simulink model "LKAS_AutoSave_DF_20220421_1805_SW62"  (R2018b)
settings: Solver=FixedStepDiscrete  StartTime=0.0  StopTime=10.0  FixedStep=0.01  RelTol=1e-3
model workspace (MAT data in the model file):
  MCOS : class17 (value not decoded)
  MCOS : class17 (value not decoded)
  MCOS : class17 (value not decoded)
  MCOS : class17 (value not decoded)
  MCOS : class17 (value not decoded)
  MCOS : class17 (value not decoded)
  MCOS : class17 (value not decoded)
  MCOS : class17 (value not decoded)
  MCOS : class17 (value not decoded)
  MCOS : class17 (value not decoded)
  MCOS : class17 (value not decoded)
  MCOS : class17 (value not decoded)
  MCOS : class17 (value not decoded)
  MCOS : class17 (value not decoded)
  MCOS : class17 (value not decoded)
  MCOS : class17 (value not decoded)
  MCOS : class17 (value not decoded)
  MCOS : class17 (value not decoded)
  MCOS : class17 (value not decoded)
  MCOS : class17 (value not decoded)
  MCOS : class17 (value not decoded)
  MCOS : class17 (value not decoded)
  MCOS : class17 (value not decoded)
  MCOS : class17 (value not decoded)
  MCOS : class17 (value not decoded)
  MCOS : class17 (value not decoded)
  MCOS : class17 (value not decoded)
  MCOS : class17 (value not decoded)
  MCOS : class17 (value not decoded)
  MCOS : class17 (value not decoded)
  MCOS : class17 (value not decoded)
  MCOS : class17 (value not decoded)
  MCOS : class17 (value not decoded)
  MCOS : class17 (value not decoded)
  MCOS : class17 (value not decoded)
  MCOS : class17 (value not decoded)
  MCOS : class17 (value not decoded)
  MCOS : class17 (value not decoded)
  MCOS : class17 (value not decoded)
  MCOS : class17 (value not decoded)
  MCOS : class17 (value not decoded)
  MCOS : class17 (value not decoded)
  MCOS : class17 (value not decoded)
  MCOS : class17 (value not decoded)
  MCOS : class17 (value not decoded)
  MCOS : class17 (value not decoded)
  MCOS : class17 (value not decoded)
  MCOS : class17 (value not decoded)
  MCOS : class17 (value not decoded)
  MCOS : class17 (value not decoded)
  MCOS : class17 (value not decoded)
  MCOS : class17 (value not decoded)
  MCOS : class17 (value not decoded)
  MCOS : class17 (value not decoded)
  MCOS : class17 (value not decoded)
  MCOS : class17 (value not decoded)
  MCOS : class17 (value not decoded)
  MCOS : class17 (value not decoded)
  MCOS : class17 (value not decoded)
  MCOS : class17 (value not decoded)
  MCOS : class17 (value not decoded)
  MCOS : class17 (value not decoded)
  MCOS : class17 (value not decoded)
  MCOS : class17 (value not decoded)
  MCOS : class17 (value not decoded)
  MCOS : class17 (value not decoded)
  MCOS : class17 (value not decoded)
  MCOS : class17 (value not decoded)
  MCOS : class17 (value not decoded)
  MCOS : class17 (value not decoded)
  MCOS : class17 (value not decoded)
  MCOS : class17 (value not decoded)
  MCOS : class17 (value not decoded)
  MCOS : class17 (value not decoded)
  MCOS : class17 (value not decoded)
  MCOS : class17 (value not decoded)
  MCOS : class17 (value not decoded)
  MCOS : class17 (value not decoded)
  MCOS : class17 (value not decoded)
  MCOS : class17 (value not decoded)
  MCOS : class17 (value not decoded)
  MCOS : class17 (value not decoded)
  MCOS : class17 (value not decoded)
  MCOS : class17 (value not decoded)
  MCOS : class17 (value not decoded)
  MCOS : class17 (value not decoded)
  MCOS : class17 (value not decoded)
  MCOS : class17 (value not decoded)
  MCOS : class17 (value not decoded)
  MCOS : class17 (value not decoded)
  MCOS : class17 (value not decoded)
  MCOS : class17 (value not decoded)
  MCOS : class17 (value not decoded)
  MCOS : class17 (value not decoded)
  MCOS : class17 (value not decoded)
  MCOS : class17 (value not decoded)
  MCOS : class17 (value not decoded)
  MCOS : class17 (value not decoded)
  MCOS : class17 (value not decoded)
  MCOS : class17 (value not decoded)
  MCOS : class17 (value not decoded)
  MCOS : class17 (value not decoded)
  MCOS : class17 (value not decoded)
  MCOS : class17 (value not decoded)
  MCOS : class17 (value not decoded)
  MCOS : class17 (value not decoded)
  MCOS : class17 (value not decoded)
  MCOS : class17 (value not decoded)
  MCOS : class17 (value not decoded)
  MCOS : class17 (value not decoded)
undefined symbols (not defined in the file): LKA_CarWidth, LKA_SampleTime, LKA_StrRatio_C, LKA_Veh2CamL_C, LKA_Veh2CamW_C, LKA_WhlBaseL_C, LL_CompHdAg_C, LL_CompSWA_C, LL_CrvtPrvwT_C, LL_DesDvt_C, LL_DvtComp_C, LL_DvtPrvwT_C, LL_DvtSpdDet_vDvtSpdMin_C, LL_HandsOff_ExitTime, LL_HandsOff_TextTime, LL_HandsOff_WarnTime, LL_HdAgExT_C, LL_HdAgPrvwT_C, LL_LAccMax_C, LL_LAccRMax_C, LL_LDW_EarliestWarnLine_C, LL_LDW_LatestWarnLine_C, LL_LDWS_SUPPRESS_HEADING, LL_LFClb_TFC_FfCtlRatio_C, LL_LFClb_TFC_KdBalance_C, LL_LFClb_TFC_KdMaxSWA_C, LL_LFClb_TFC_KdV1_C, LL_LFClb_TFC_KdV2_C, LL_LFClb_TFC_KdVehSpdLwr_C, LL_LFClb_TFC_KdVehSpdUpr_C, LL_LFClb_TFC_Ki_C, LL_LFClb_TFC_KiMaxSWA_C, LL_LFClb_TFC_Kp_C, LL_LFClb_TFC_KpKlat_C, LL_LFClb_TFC_KpV1_C, LL_LFClb_TFC_KpV2_C, LL_LFClb_TFC_KpVehSpdLwr_C, LL_LFClb_TFC_KpVehSpdUpr_C, LL_LFClb_TFC_PrvwT_C, LL_LKA_EarliestWarnLine_C, LL_LKA_EnableLine_DvtMax, LL_LKA_EnableLine_DvtMin, LL_LKA_EnableLine_Max, LL_LKA_LatestWarnLine_C, LL_LKAExPrcs_ExitC0Dvt, LL_LKAExPrcs_ExitC0Swt, LL_LKAExPrcs_tiExitDelayTime3, LL_LKAExPrcs_tiExitTime1, LL_LKAExPrcs_tiExitTime2, LL_LKAExPrcs_tiExitTime3, LL_LKAS_OUT_OF_CONTROL_LAT_VEL, LL_LKAS_OUT_OF_CONTROL_TTLC, LL_LKASWASyn_M0, LL_LKASWASyn_M1, LL_LKASWASyn_M2, LL_LKASWASyn_M3D, LL_LKASWASyn_M3K_DT, LL_LKASWASyn_M3K_MSD, LL_LKASWASyn_M4K, LL_LKASWASyn_SWAaddMax ... (+51)
libraries: simulink x241, canmsglib x6, dspstat3 x3, simulink_extras x1
(part 2 of 18)

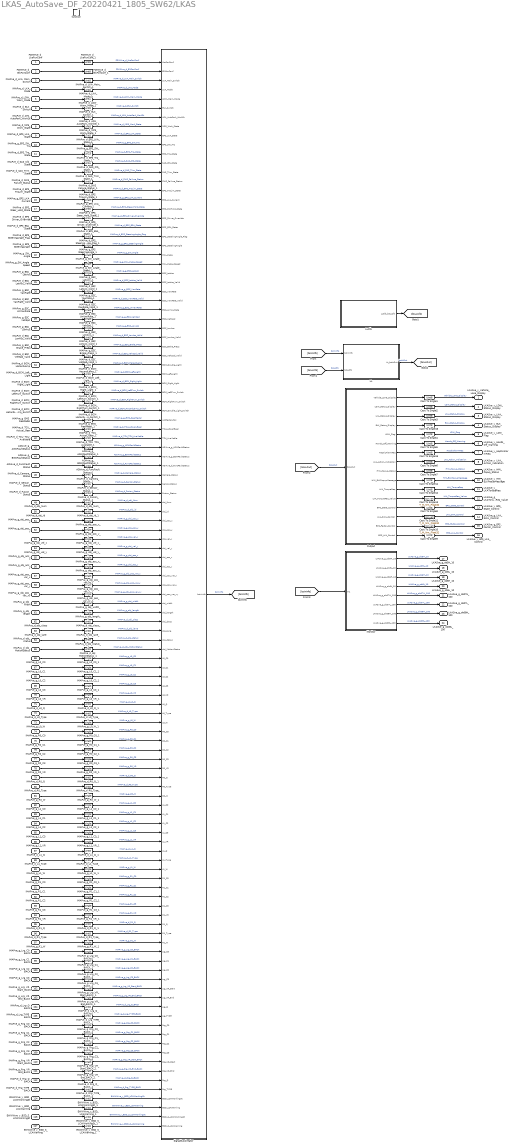
== system LKAS_AutoSave_DF_20220421_1805_SW62/LKAS ==
  FDMMve_d_LkaFcnConf : Inport
  FDMMve_d_ElkFcnConf : Inport  Port=2
  IMAPve_d_LKA_Main_Switch : Inport  Port=3
  IMAPve_d_LKA_Mode : Inport  Port=4
  IMAPve_d_LDW_Warn_Mode : Inport  Port=5
  IMAPve_d_ELK_Switch : Inport  Port=6
  IMAPve_d_APA_AutoPark_WorkSt : Inport  Port=7
  IMAPve_d_MP5_Work_State : Inport  Port=8
  IMAPve_d_EPS_LKA_State : Inport  Port=9
  IMAPve_g_EPS_SW_Trq : Inport  Port=10
  IMAPve_d_EPS_Trq_State : Inport  Port=11
  IMAPve_d_SAS_Clb_State : Inport  Port=12
  IMAPve_d_SAS_Trim_State : Inport  Port=13
  IMAPve_d_SWS_Failure_Status : Inport  Port=14
  IMAPve_d_EPS_TrqLim_State : Inport  Port=15
  IMAPve_g_EPS_LKA_Current : Inport  Port=16
  IMAPve_d_EPS_Steer_Hold_State : Inport  Port=17
  IMAPve_d_EPS_Driver_Override : Inport  Port=18
  IMAPve_d_EPS_ESA_State : Inport  Port=19
  IMAPve_d_EPS_SteeringAngle_Flag : Inport  Port=20
  IMAPve_g_EPS_SteeringAngle : Inport  Port=21
  IMAPve_g_SW_Angle : Inport  Port=22
  IMAPve_g_SW_Angle_Speed : Inport  Port=23
  IMAPve_g_ESC_LatAcc : Inport  Port=24
  IMAPve_d_ESC_LatAcc_Valid : Inport  Port=25
  IMAPve_g_ESC_YawRate : Inport  Port=26
  IMAPve_d_ESC_YawRate_Valid : Inport  Port=27
  IMAPve_g_ESC_UnYawRate : Inport  Port=28
  IMAPve_g_ESC_VehSpd : Inport  Port=29
  IMAPve_g_ESC_LonAcc : Inport  Port=30
  IMAPve_d_ESC_LonAcc_Valid : Inport  Port=31
  IMAPve_g_ESC_Brake_Press : Inport  Port=32
  IMAPve_d_ESC_VehSpd_Valid : Inport  Port=33
  IMAPve_d_BCM_HazardLamp : Inport  Port=34
  IMAPve_d_BCM_Left_Light : Inport  Port=35
  IMAPve_d_BCM_Right_Light : Inport  Port=36
  IMAPve_d_BCM_LeftTurn_Switch : Inport  Port=37
  IMAPve_d_BCM_RightTurn_Switch : Inport  Port=38
  IMAPve_d_BCM_HazardLamp_Switch : Inport  Port=39
  IMAPve_g_EMS_RealPedal : Inport  Port=40
  IMAPve_d_TCU_Actual_Gear : Inport  Port=41
  IMAPve_d_TCU_TCU_Available : Inport  Port=42
  ADIAve_g_ASWFaultStatus : Inport  Port=43
  ADIAve_g_BSWFaultStatus : Inport  Port=44
  ADIAve_d_FuncFaultStatus : Inport  Port=45
  IMAPve_d_Camera_Status : Inport  Port=46
  IMAPve_d_Sensor_Status : Inport  Port=47
  IMAPve_d_Fusion_Status : Inport  Port=48
  IMAPve_d_obj_Num : Inport  Port=49
  IMAPva_d_obj_id : Inport  Port=50
  IMAPva_g_obj_pos_x : Inport  Port=51
  IMAPva_g_obj_pos_y : Inport  Port=52
  IMAPva_g_obj_vel_x : Inport  Port=53
  IMAPva_g_obj_vel_y : Inport  Port=54
  IMAPva_g_obj_acc_x : Inport  Port=55
  IMAPva_g_obj_acc_y : Inport  Port=56
  IMAPva_g_obj_pos_var_x : Inport  Port=57
  IMAPva_g_obj_pos_var_y : Inport  Port=58
  IMAPva_g_obj_pos_var_xy : Inport  Port=59
  IMAPva_g_obj_width : Inport  Port=60
  IMAPva_g_obj_length : Inport  Port=61
  IMAPva_d_obj_class : Inport  Port=62
  IMAPva_d_obj_lane : Inport  Port=63
  IMAPva_d_obj_status : Inport  Port=64
  IMAPva_d_obj_MotionStatus : Inport  Port=65
  IMAPve_g_L0_C0 : Inport  Port=66
  IMAPve_g_L0_C1 : Inport  Port=67
  IMAPve_g_L0_C2 : Inport  Port=68
  IMAPve_g_L0_C3 : Inport  Port=69
  IMAPve_g_L0_VR : Inport  Port=70
  IMAPve_d_L0_Q : Inport  Port=71
  IMAPve_d_L0_Type : Inport  Port=72
  IMAPve_g_L0_W : Inport  Port=73
  IMAPve_g_R0_C0 : Inport  Port=74
  IMAPve_g_R0_C1 : Inport  Port=75
  IMAPve_g_R0_C2 : Inport  Port=76
  IMAPve_g_R0_C3 : Inport  Port=77
  IMAPve_g_R0_VR : Inport  Port=78
  IMAPve_d_R0_Q : Inport  Port=79
  IMAPve_d_R0_Type : Inport  Port=80
  IMAPve_g_R0_W : Inport  Port=81
  IMAPve_g_L1_C0 : Inport  Port=82
  IMAPve_g_L1_C1 : Inport  Port=83
  IMAPve_g_L1_C2 : Inport  Port=84
  IMAPve_g_L1_C3 : Inport  Port=85
  IMAPve_g_L1_VR : Inport  Port=86
  IMAPve_d_L1_Q : Inport  Port=87
  IMAPve_d_L1_Type : Inport  Port=88
  IMAPve_g_L1_W : Inport  Port=89
  IMAPve_g_R1_C0 : Inport  Port=90
  IMAPve_g_R1_C1 : Inport  Port=91
  IMAPve_g_R1_C2 : Inport  Port=92
  IMAPve_g_R1_C3 : Inport  Port=93
  IMAPve_g_R1_VR : Inport  Port=94
  IMAPve_d_R1_Q : Inport  Port=95
  IMAPve_d_R1_Type : Inport  Port=96
  IMAPve_g_R1_W : Inport  Port=97
  IMAPve_g_Lrg_C0_BACK : Inport  Port=98
  IMAPve_g_Lrg_C1_BACK : Inport  Port=99
  IMAPve_g_Lrg_C2_BACK : Inport  Port=100
  IMAPve_g_Lrg_C3_BACK : Inport  Port=101
  IMAPve_g_Lrg_VR_Start_BACK : Inport  Port=102
  IMAPve_g_Lrg_VR_End_BACK : Inport  Port=103
  IMAPve_d_Lrg_Q_BACK : Inport  Port=104
  IMAPve_d_Lrg_TYPE_BACK : Inport  Port=105
  IMAPve_g_Rrg_C0_BACK : Inport  Port=106
  IMAPve_g_Rrg_C1_BACK : Inport  Port=107
  IMAPve_g_Rrg_C2_BACK : Inport  Port=108
  IMAPve_g_Rrg_C3_BACK : Inport  Port=109
  IMAPve_g_Rrg_VR_Start_BACK : Inport  Port=110
  IMAPve_g_Rrg_VR_End_BACK : Inport  Port=111
  IMAPve_d_Rrg_Q_BACK : Inport  Port=112
  IMAPve_d_Rrg_TYPE_BACK : Inport  Port=113
  EWWWve_y_BSD_LCWWorkingSt : Inport  Port=114
  EWWWve_y_BSD_LCAWarning : Inport  Port=115
  EWWWve_y_BSD_S_LCWWorkingSt : Inport  Port=116
  EWWWve_y_BSD_S_LCAWarning : Inport  Port=117
  function : TriggerPort  TriggerType=function-call  VariantControl=Variant  SampleTimeType=periodic  SampleTime=-1
  ADIAve_d_FuncFaultStatus_1 : DataTypeConversion  OutDataTypeStr=uint8
  ADIAve_g_ASWFaultStatus_1 : DataTypeConversion  OutDataTypeStr=single
  ADIAve_g_BSWFaultStatus_1 : DataTypeConversion  OutDataTypeStr=single
  Cast To Single{1..9,12,14..16} (13 alike) : DataTypeConversion  OutDataTypeStr=UInt8
  Cast To Single10 : DataTypeConversion  OutDataTypeStr=T_M_Nm_Float32
  Cast To Single11 : DataTypeConversion  OutDataTypeStr=T_M_Nm_Float32
  Cast To Single13 : DataTypeConversion  OutDataTypeStr=T_M_Nm_Float32
  EWWWve_y_BSD_LCAWarning_1 : DataTypeConversion  OutDataTypeStr=uint8
  EWWWve_y_BSD_LCWWorkingSt_1 : DataTypeConversion  OutDataTypeStr=uint8
  EWWWve_y_BSD_S_LCAWarning_1 : DataTypeConversion  OutDataTypeStr=uint8
  EWWWve_y_BSD_S_LCWWorkingSt_1 : DataTypeConversion  OutDataTypeStr=uint8
  FDMMve_d_ElkFcnConf_1 : DataTypeConversion  OutDataTypeStr=uint8
  FDMMve_d_LkaFcnConf_1 : DataTypeConversion  OutDataTypeStr=uint8
  IMAPva_d_obj_MotionStatus_1 : DataTypeConversion  OutDataTypeStr=uint8
  IMAPva_d_obj_class_1 : DataTypeConversion  OutDataTypeStr=uint8
  IMAPva_d_obj_id_1 : DataTypeConversion  OutDataTypeStr=uint8
  IMAPva_d_obj_lane_1 : DataTypeConversion  OutDataTypeStr=uint8
  IMAPva_d_obj_status_1 : DataTypeConversion  OutDataTypeStr=uint8
  IMAPva_g_obj_acc_x_1 : DataTypeConversion  OutDataTypeStr=single
  IMAPva_g_obj_acc_y_1 : DataTypeConversion  OutDataTypeStr=single
  IMAPva_g_obj_length_1 : DataTypeConversion  OutDataTypeStr=single
  IMAPva_g_obj_pos_var_x_1 : DataTypeConversion  OutDataTypeStr=single
  IMAPva_g_obj_pos_var_xy_1 : DataTypeConversion  OutDataTypeStr=single
  IMAPva_g_obj_pos_var_y_1 : DataTypeConversion  OutDataTypeStr=single
  IMAPva_g_obj_pos_x_1 : DataTypeConversion  OutDataTypeStr=single
  IMAPva_g_obj_pos_y_1 : DataTypeConversion  OutDataTypeStr=single
  IMAPva_g_obj_vel_x_1 : DataTypeConversion  OutDataTypeStr=single
  IMAPva_g_obj_vel_y_1 : DataTypeConversion  OutDataTypeStr=single
  IMAPva_g_obj_width_1 : DataTypeConversion  OutDataTypeStr=single
  IMAPve_d_APA_AutoPark_WorkSt_1 : DataTypeConversion  OutDataTypeStr=uint8
  IMAPve_d_BCM_HazardLamp_1 : DataTypeConversion  OutDataTypeStr=uint8
  IMAPve_d_BCM_HazardLamp_Switch_1 : DataTypeConversion  OutDataTypeStr=uint8
  IMAPve_d_BCM_LeftTurn_Switch_1 : DataTypeConversion  OutDataTypeStr=uint8
  IMAPve_d_BCM_Left_Light_1 : DataTypeConversion  OutDataTypeStr=uint8
  IMAPve_d_BCM_RightTurn_Switch_1 : DataTypeConversion  OutDataTypeStr=uint8
  IMAPve_d_BCM_Right_Light_1 : DataTypeConversion  OutDataTypeStr=uint8
  IMAPve_d_Camera_Status_1 : DataTypeConversion  OutDataTypeStr=uint8
  IMAPve_d_ELK_Switch_1 : DataTypeConversion  OutDataTypeStr=uint8
  IMAPve_d_EPS_Driver_Override_1 : DataTypeConversion  OutDataTypeStr=uint8
  IMAPve_d_EPS_ESA_State_1 : DataTypeConversion  OutDataTypeStr=uint8
  IMAPve_d_EPS_LKA_State_1 : DataTypeConversion  OutDataTypeStr=uint8
  IMAPve_d_EPS_Steer_Hold_State_1 : DataTypeConversion  OutDataTypeStr=uint8
  IMAPve_d_EPS_SteeringAngle_Flag_1 : DataTypeConversion  OutDataTypeStr=uint8
  IMAPve_d_EPS_TrqLim_State_1 : DataTypeConversion  OutDataTypeStr=uint8
  IMAPve_d_EPS_Trq_State_1 : DataTypeConversion  OutDataTypeStr=uint8
  IMAPve_d_ESC_LatAcc_Valid_1 : DataTypeConversion  OutDataTypeStr=uint8
  IMAPve_d_ESC_LonAcc_Valid_1 : DataTypeConversion  OutDataTypeStr=uint8
  IMAPve_d_ESC_VehSpd_Valid_1 : DataTypeConversion  OutDataTypeStr=uint8
  IMAPve_d_ESC_YawRate_Valid_1 : DataTypeConversion  OutDataTypeStr=uint8
  IMAPve_d_Fusion_Status_1 : DataTypeConversion  OutDataTypeStr=uint8
  IMAPve_d_L0_Q_1 : DataTypeConversion  OutDataTypeStr=uint8
  IMAPve_d_L0_Type_1 : DataTypeConversion  OutDataTypeStr=uint8
  IMAPve_d_L1_Q_1 : DataTypeConversion  OutDataTypeStr=uint8
  IMAPve_d_L1_Type_1 : DataTypeConversion  OutDataTypeStr=uint8
  IMAPve_d_LDW_Warn_Mode_1 : DataTypeConversion  OutDataTypeStr=uint8
  IMAPve_d_LKA_Main_Switch_1 : DataTypeConversion  OutDataTypeStr=uint8
  IMAPve_d_LKA_Mode_1 : DataTypeConversion  OutDataTypeStr=uint8
  IMAPve_d_Lrg_Q_BACK_1 : DataTypeConversion  OutDataTypeStr=uint8
  IMAPve_d_Lrg_TYPE_BACK_1 : DataTypeConversion  OutDataTypeStr=uint8
  IMAPve_d_MP5_Work_State_1 : DataTypeConversion  OutDataTypeStr=uint8
  IMAPve_d_R0_Q_1 : DataTypeConversion  OutDataTypeStr=uint8
  IMAPve_d_R0_Type_1 : DataTypeConversion  OutDataTypeStr=uint8
  IMAPve_d_R1_Q_1 : DataTypeConversion  OutDataTypeStr=uint8
  IMAPve_d_R1_Type_1 : DataTypeConversion  OutDataTypeStr=uint8
  IMAPve_d_Rrg_Q_BACK_1 : DataTypeConversion  OutDataTypeStr=uint8
  IMAPve_d_Rrg_TYPE_BACK_1 : DataTypeConversion  OutDataTypeStr=uint8
  IMAPve_d_SAS_Clb_State_1 : DataTypeConversion  OutDataTypeStr=uint8
  IMAPve_d_SAS_Trim_State_1 : DataTypeConversion  OutDataTypeStr=uint8
  IMAPve_d_SWS_Failure_Status_1 : DataTypeConversion  OutDataTypeStr=uint8
  IMAPve_d_Sensor_Status_1 : DataTypeConversion  OutDataTypeStr=uint8
  IMAPve_d_TCU_Actual_Gear_1 : DataTypeConversion  OutDataTypeStr=uint8
  IMAPve_d_TCU_TCU_Available_1 : DataTypeConversion  OutDataTypeStr=uint8
  IMAPve_d_obj_Num_1 : DataTypeConversion  OutDataTypeStr=uint8
  IMAPve_g_EMS_RealPedal_1 : DataTypeConversion  OutDataTypeStr=single
  IMAPve_g_EPS_LKA_Current_1 : DataTypeConversion  OutDataTypeStr=single
  IMAPve_g_EPS_SW_Trq_1 : DataTypeConversion  OutDataTypeStr=single
  IMAPve_g_EPS_SteeringAngle_1 : DataTypeConversion  OutDataTypeStr=single
  IMAPve_g_ESC_Brake_Press_1 : DataTypeConversion  OutDataTypeStr=single
  IMAPve_g_ESC_LatAcc_1 : DataTypeConversion  OutDataTypeStr=single
  IMAPve_g_ESC_LonAcc_1 : DataTypeConversion  OutDataTypeStr=single
  IMAPve_g_ESC_UnYawRate_1 : DataTypeConversion  OutDataTypeStr=single
  IMAPve_g_ESC_VehSpd_1 : DataTypeConversion  OutDataTypeStr=single
  IMAPve_g_ESC_YawRate_1 : DataTypeConversion  OutDataTypeStr=single
  IMAPve_g_L0_C0_1 : DataTypeConversion  OutDataTypeStr=single
  IMAPve_g_L0_C1_1 : DataTypeConversion  OutDataTypeStr=single
  IMAPve_g_L0_C2_1 : DataTypeConversion  OutDataTypeStr=single
  IMAPve_g_L0_C3_1 : DataTypeConversion  OutDataTypeStr=single
  IMAPve_g_L0_VR_1 : DataTypeConversion  OutDataTypeStr=single
  IMAPve_g_L0_W_1 : DataTypeConversion  OutDataTypeStr=single
  IMAPve_g_L1_C0_1 : DataTypeConversion  OutDataTypeStr=single
  IMAPve_g_L1_C1_1 : DataTypeConversion  OutDataTypeStr=single
  IMAPve_g_L1_C2_1 : DataTypeConversion  OutDataTypeStr=single
  IMAPve_g_L1_C3_1 : DataTypeConversion  OutDataTypeStr=single
  IMAPve_g_L1_VR_1 : DataTypeConversion  OutDataTypeStr=single
  IMAPve_g_L1_W_1 : DataTypeConversion  OutDataTypeStr=single
  IMAPve_g_Lrg_C0_BACK_1 : DataTypeConversion  OutDataTypeStr=single
  IMAPve_g_Lrg_C1_BACK_1 : DataTypeConversion  OutDataTypeStr=single
  IMAPve_g_Lrg_C2_BACK_1 : DataTypeConversion  OutDataTypeStr=single
  IMAPve_g_Lrg_C3_BACK_1 : DataTypeConversion  OutDataTypeStr=single
  IMAPve_g_Lrg_VR_End_BACK_1 : DataTypeConversion  OutDataTypeStr=single
  IMAPve_g_Lrg_VR_Start_BACK_1 : DataTypeConversion  OutDataTypeStr=single
  IMAPve_g_R0_C0_1 : DataTypeConversion  OutDataTypeStr=single
  IMAPve_g_R0_C1_1 : DataTypeConversion  OutDataTypeStr=single
  IMAPve_g_R0_C2_1 : DataTypeConversion  OutDataTypeStr=single
  IMAPve_g_R0_C3_1 : DataTypeConversion  OutDataTypeStr=single
  IMAPve_g_R0_VR_1 : DataTypeConversion  OutDataTypeStr=single
  IMAPve_g_R0_W_1 : DataTypeConversion  OutDataTypeStr=single
  IMAPve_g_R1_C0_1 : DataTypeConversion  OutDataTypeStr=single
  IMAPve_g_R1_C1_1 : DataTypeConversion  OutDataTypeStr=single
  IMAPve_g_R1_C2_1 : DataTypeConversion  OutDataTypeStr=single
  IMAPve_g_R1_C3_1 : DataTypeConversion  OutDataTypeStr=single
  IMAPve_g_R1_VR_1 : DataTypeConversion  OutDataTypeStr=single
  IMAPve_g_R1_W_1 : DataTypeConversion  OutDataTypeStr=single
  IMAPve_g_Rrg_C0_BACK_1 : DataTypeConversion  OutDataTypeStr=single
  IMAPve_g_Rrg_C1_BACK_1 : DataTypeConversion  OutDataTypeStr=single
  IMAPve_g_Rrg_C2_BACK_1 : DataTypeConversion  OutDataTypeStr=single
  IMAPve_g_Rrg_C3_BACK_1 : DataTypeConversion  OutDataTypeStr=single
  IMAPve_g_Rrg_VR_End_BACK_1 : DataTypeConversion  OutDataTypeStr=single
  IMAPve_g_Rrg_VR_Start_BACK_1 : DataTypeConversion  OutDataTypeStr=single
  IMAPve_g_SW_Angle_1 : DataTypeConversion  OutDataTypeStr=single
  IMAPve_g_SW_Angle_Speed_1 : DataTypeConversion  OutDataTypeStr=single
  LL : Subsystem
  LLClb : Subsystem
  Monitor : Subsystem  SystemSampleTime=0.01
  Output : Subsystem
  SignalBusCreator : Subsystem
  LKASve_y_Vehicle_Lane_Display : Outport
  LKASve_y_LDW_Status_Display : Outport  Port=2
  LKASve_y_LKA_Status_Display : Outport  Port=3
  LKASve_y_ELK_Status_Display : Outport  Port=4
  LKASve_y_LDW_Flag : Outport  Port=5
  LKASve_y_Hands_Off_Warning : Outport  Port=6
  LKASve_y_HapticAlarmReq : Outport  Port=7
  LKASve_y_LKA_Action_Indication : Outport  Port=8
  LKASve_y_HMI_Popup_Status : Outport  Port=9
  LKASve_y_HMI_ELKPopupMessage : Outport  Port=10
  LKASve_y_LKATorqueReq : Outport  Port=11
  LKASve_g_LKATorqueReq_Value : Outport  Port=12
  LKASve_y_EPS_State_Control : Outport  Port=13
  LKASve_g_LKA_SWA_Control : Outport  Port=14
  LKASve_g_EPS_Factor_Control : Outport  Port=15
  LKASve_y_EPS_LKA_Control : Outport  Port=16
  LKASve_g_ob5H_10 : Outport  Port=17
  LKASve_g_ob5L_10 : Outport  Port=18
  LKASve_g_ob6H_10 : Outport  Port=19
  LKASve_g_ob6L_10 : Outport  Port=20
  LKASve_g_ob07H_100 : Outport  Port=21
  LKASve_g_ob07L_100 : Outport  Port=22
  LKASve_g_ob08H_100 : Outport  Port=23
  LKASve_g_ob08L_100 : Outport  Port=24
  wires:
  [bsInInfo] -> Monitor/1(In1)
  Output/4(ELK_Status_Display) -> Cast To Single16/1
  Output/7(HapticAlarmReq) -> Cast To Single15/1
  Output/10(HMI_ELKPopupMessage) -> Cast To Single14/1
  Output/2(LDW_Status_Display) -> Cast To Single2/1
  Output/6(Hands_Off_Warning) -> Cast To Single5/1
  [bsLLClb] -> LL/2(bsLLClb)  "bsLLClb"
  Output/16(EPS_LKA_Control) -> Cast To Single9/1
  LLClb/1(LLClb_bsLLClb) -> [bsLLClb]
  Cast To Single7/1 -> LKASve_y_HMI_Popup_Status/1  "HMI_Popup_Status"
  Cast To Single3/1 -> LKASve_y_LKA_Status_Display/1  "LKA_Status_Display"
  Cast To Single10/1 -> LKASve_g_EPS_Factor_Control/1  "EPS_Factor_Control"
  Output/8(LKA_Action_Indication) -> Cast To Single6/1
  [bsInInfo] -> LL/1(bsInInfo)  "bsInInfo"
  Cast To Single8/1 -> LKASve_y_EPS_State_Control/1  "EPS_State_Control"
  Output/3(LKA_Status_Display) -> Cast To Single3/1
  Output/1(Vehicle_Lane_Display) -> Cast To Single1/1
  Output/13(EPS_State_Control) -> Cast To Single8/1
  Output/12(LKA_TorqueReq_Value) -> Cast To Single13/1
  Output/11(LKA_TorqueReq) -> Cast To Single12/1
  Cast To Single6/1 -> LKASve_y_LKA_Action_Indication/1  "LKA_Action_Indication"
  Output/15(EPS_Factor_Control) -> Cast To Single10/1
  Output/5(LDW_Flag) -> Cast To Single4/1
  Cast To Single4/1 -> LKASve_y_LDW_Flag/1  "LDW_Flag"
  Cast To Single11/1 -> LKASve_g_LKA_SWA_Control/1  "LKA_SWA_Control"
  LL/1(LL_bsLLOut) -> [bsLLOut]  "bsLLOut"
  Cast To Single5/1 -> LKASve_y_Hands_Off_Warning/1  "Hands_Off_Warning"
  Cast To Single12/1 -> LKASve_y_LKATorqueReq/1  "LKA_TorqueReq"
  Cast To Single13/1 -> LKASve_g_LKATorqueReq_Value/1  "LKA_TorqueReq_Value"
  SignalBusCreator/1(bsInInfo) -> [bsInInfo]  "bsInInfo"
  Cast To Single9/1 -> LKASve_y_EPS_LKA_Control/1  "EPS_LKA_Control"
  Cast To Single1/1 -> LKASve_y_Vehicle_Lane_Display/1  "Vehicle_Lane_Display"
  Cast To Single2/1 -> LKASve_y_LDW_Status_Display/1  "LDW_Status_Display"
  Output/9(HMI_Popup_Status) -> Cast To Single7/1
  Output/14(LKA_SWA_Control) -> Cast To Single11/1
  [bsLLOut] -> Output/1(bsLLOut)  "bsLLOut"
  Monitor/8(LKASve_g_ob08L_100) -> LKASve_g_ob08L_100/1  "LKASve_g_ob08L_100"
  Monitor/7(LKASve_g_ob08H_100) -> LKASve_g_ob08H_100/1  "LKASve_g_ob08H_100"
  Monitor/6(LKASve_g_ob07L_100) -> LKASve_g_ob07L_100/1  "LKASve_g_ob07L_100"
  Monitor/5(LKASve_g_ob07H_100) -> LKASve_g_ob07H_100/1  "LKASve_g_ob07H_100"
  Monitor/4(LKASve_g_ob6L_10) -> LKASve_g_ob6L_10/1  "LKASve_g_ob6L_10"
  Monitor/3(LKASve_g_ob6H_10) -> LKASve_g_ob6H_10/1  "LKASve_g_ob6H_10"
  Monitor/2(LKASve_g_ob5L_10) -> LKASve_g_ob5L_10/1  "LKASve_g_ob5L_10"
  Monitor/1(LKASve_g_ob5H_10) -> LKASve_g_ob5H_10/1  "LKASve_g_ob5H_10"
  Cast To Single14/1 -> LKASve_y_HMI_ELKPopupMessage/1  "HMI_ELKPopupMessage"
  Cast To Single15/1 -> LKASve_y_HapticAlarmReq/1  "HapticAlarmReq"
  Cast To Single16/1 -> LKASve_y_ELK_Status_Display/1  "ELK_Status_Display"
  EWWWve_y_BSD_S_LCAWarning_1/1 -> SignalBusCreator/117(BSD_S_LCAWarning)  "EWWWve_y_BSD_S_LCAWarning"
  EWWWve_y_BSD_S_LCAWarning/1 -> EWWWve_y_BSD_S_LCAWarning_1/1
  EWWWve_y_BSD_S_LCWWorkingSt_1/1 -> SignalBusCreator/116(BSD_S_LCWWorkingSt)  "EWWWve_y_BSD_S_LCWWorkingSt"
  EWWWve_y_BSD_S_LCWWorkingSt/1 -> EWWWve_y_BSD_S_LCWWorkingSt_1/1
  EWWWve_y_BSD_LCAWarning_1/1 -> SignalBusCreator/115(BSD_LCAWarning)  "EWWWve_y_BSD_LCAWarning"
  EWWWve_y_BSD_LCAWarning/1 -> EWWWve_y_BSD_LCAWarning_1/1
  EWWWve_y_BSD_LCWWorkingSt_1/1 -> SignalBusCreator/114(BSD_LCWWorkingSt)  "EWWWve_y_BSD_LCWWorkingSt"
  EWWWve_y_BSD_LCWWorkingSt/1 -> EWWWve_y_BSD_LCWWorkingSt_1/1
  IMAPve_d_Rrg_TYPE_BACK_1/1 -> SignalBusCreator/113(Rrg_TYPE)  "IMAPve_d_Rrg_TYPE_BACK"
  IMAPve_d_Rrg_TYPE_BACK/1 -> IMAPve_d_Rrg_TYPE_BACK_1/1
  IMAPve_d_Rrg_Q_BACK_1/1 -> SignalBusCreator/112(Rrg_Q)  "IMAPve_d_Rrg_Q_BACK"
  IMAPve_d_Rrg_Q_BACK/1 -> IMAPve_d_Rrg_Q_BACK_1/1
  IMAPve_g_Rrg_VR_End_BACK_1/1 -> SignalBusCreator/111(Rrg_VR_End)  "IMAPve_g_Rrg_VR_End_BACK"
  IMAPve_g_Rrg_VR_End_BACK/1 -> IMAPve_g_Rrg_VR_End_BACK_1/1
  IMAPve_g_Rrg_VR_Start_BACK_1/1 -> SignalBusCreator/110(Rrg_VR_Start)  "IMAPve_g_Rrg_VR_Start_BACK"
  IMAPve_g_Rrg_VR_Start_BACK/1 -> IMAPve_g_Rrg_VR_Start_BACK_1/1
  IMAPve_g_Rrg_C3_BACK_1/1 -> SignalBusCreator/109(Rrg_C3)  "IMAPve_g_Rrg_C3_BACK"
  IMAPve_g_Rrg_C3_BACK/1 -> IMAPve_g_Rrg_C3_BACK_1/1
  IMAPve_g_Rrg_C2_BACK_1/1 -> SignalBusCreator/108(Rrg_C2)  "IMAPve_g_Rrg_C2_BACK"
  IMAPve_g_Rrg_C2_BACK/1 -> IMAPve_g_Rrg_C2_BACK_1/1
  IMAPve_g_Rrg_C1_BACK_1/1 -> SignalBusCreator/107(Rrg_C1)  "IMAPve_g_Rrg_C1_BACK"
  IMAPve_g_Rrg_C1_BACK/1 -> IMAPve_g_Rrg_C1_BACK_1/1
  IMAPve_g_Rrg_C0_BACK_1/1 -> SignalBusCreator/106(Rrg_C0)  "IMAPve_g_Rrg_C0_BACK"
  IMAPve_g_Rrg_C0_BACK/1 -> IMAPve_g_Rrg_C0_BACK_1/1
  IMAPve_d_Lrg_TYPE_BACK_1/1 -> SignalBusCreator/105(Lrg_TYPE)  "IMAPve_d_Lrg_TYPE_BACK"
  IMAPve_d_Lrg_TYPE_BACK/1 -> IMAPve_d_Lrg_TYPE_BACK_1/1
  IMAPve_d_Lrg_Q_BACK_1/1 -> SignalBusCreator/104(Lrg_Q)  "IMAPve_d_Lrg_Q_BACK"
  IMAPve_d_Lrg_Q_BACK/1 -> IMAPve_d_Lrg_Q_BACK_1/1
  IMAPve_g_Lrg_VR_End_BACK_1/1 -> SignalBusCreator/103(Lrg_VR_End)  "IMAPve_g_Lrg_VR_End_BACK"
  IMAPve_g_Lrg_VR_End_BACK/1 -> IMAPve_g_Lrg_VR_End_BACK_1/1
  IMAPve_g_Lrg_VR_Start_BACK_1/1 -> SignalBusCreator/102(Lrg_VR_Start)  "IMAPve_g_Lrg_VR_Start_BACK"
  IMAPve_g_Lrg_VR_Start_BACK/1 -> IMAPve_g_Lrg_VR_Start_BACK_1/1
  IMAPve_g_Lrg_C3_BACK_1/1 -> SignalBusCreator/101(Lrg_C3)  "IMAPve_g_Lrg_C3_BACK"
  IMAPve_g_Lrg_C3_BACK/1 -> IMAPve_g_Lrg_C3_BACK_1/1
  IMAPve_g_Lrg_C2_BACK_1/1 -> SignalBusCreator/100(Lrg_C2)  "IMAPve_g_Lrg_C2_BACK"
  IMAPve_g_Lrg_C2_BACK/1 -> IMAPve_g_Lrg_C2_BACK_1/1
  IMAPve_g_Lrg_C1_BACK_1/1 -> SignalBusCreator/99(Lrg_C1)  "IMAPve_g_Lrg_C1_BACK"
  IMAPve_g_Lrg_C1_BACK/1 -> IMAPve_g_Lrg_C1_BACK_1/1
  IMAPve_g_Lrg_C0_BACK_1/1 -> SignalBusCreator/98(Lrg_C0)  "IMAPve_g_Lrg_C0_BACK"
  IMAPve_g_Lrg_C0_BACK/1 -> IMAPve_g_Lrg_C0_BACK_1/1
  IMAPve_g_R1_W_1/1 -> SignalBusCreator/97(R1_W)  "IMAPve_g_R1_W"
  IMAPve_g_R1_W/1 -> IMAPve_g_R1_W_1/1
  IMAPve_d_R1_Type_1/1 -> SignalBusCreator/96(R1_Type)  "IMAPve_d_R1_Type"
  IMAPve_d_R1_Type/1 -> IMAPve_d_R1_Type_1/1
  IMAPve_d_R1_Q_1/1 -> SignalBusCreator/95(R1_Q)  "IMAPve_d_R1_Q"
  IMAPve_d_R1_Q/1 -> IMAPve_d_R1_Q_1/1
  IMAPve_g_R1_VR_1/1 -> SignalBusCreator/94(R1_VR)  "IMAPve_g_R1_VR"
  IMAPve_g_R1_VR/1 -> IMAPve_g_R1_VR_1/1
  IMAPve_g_R1_C3_1/1 -> SignalBusCreator/93(R1_C3)  "IMAPve_g_R1_C3"
  IMAPve_g_R1_C3/1 -> IMAPve_g_R1_C3_1/1
  IMAPve_g_R1_C2_1/1 -> SignalBusCreator/92(R1_C2)  "IMAPve_g_R1_C2"
  IMAPve_g_R1_C2/1 -> IMAPve_g_R1_C2_1/1
  IMAPve_g_R1_C1_1/1 -> SignalBusCreator/91(R1_C1)  "IMAPve_g_R1_C1"
  IMAPve_g_R1_C1/1 -> IMAPve_g_R1_C1_1/1
  IMAPve_g_R1_C0_1/1 -> SignalBusCreator/90(R1_C0)  "IMAPve_g_R1_C0"
  IMAPve_g_R1_C0/1 -> IMAPve_g_R1_C0_1/1
  IMAPve_g_L1_W_1/1 -> SignalBusCreator/89(L1_W)  "IMAPve_g_L1_W"
  IMAPve_g_L1_W/1 -> IMAPve_g_L1_W_1/1
  IMAPve_d_L1_Type_1/1 -> SignalBusCreator/88(L1_Type)  "IMAPve_d_L1_Type"
  IMAPve_d_L1_Type/1 -> IMAPve_d_L1_Type_1/1
  IMAPve_d_L1_Q_1/1 -> SignalBusCreator/87(L1_Q)  "IMAPve_d_L1_Q"
  IMAPve_d_L1_Q/1 -> IMAPve_d_L1_Q_1/1
  IMAPve_g_L1_VR_1/1 -> SignalBusCreator/86(L1_VR)  "IMAPve_g_L1_VR"
  IMAPve_g_L1_VR/1 -> IMAPve_g_L1_VR_1/1
  IMAPve_g_L1_C3_1/1 -> SignalBusCreator/85(L1_C3)  "IMAPve_g_L1_C3"
  IMAPve_g_L1_C3/1 -> IMAPve_g_L1_C3_1/1
  IMAPve_g_L1_C2_1/1 -> SignalBusCreator/84(L1_C2)  "IMAPve_g_L1_C2"
  IMAPve_g_L1_C2/1 -> IMAPve_g_L1_C2_1/1
  IMAPve_g_L1_C1_1/1 -> SignalBusCreator/83(L1_C1)  "IMAPve_g_L1_C1"
  IMAPve_g_L1_C1/1 -> IMAPve_g_L1_C1_1/1
  IMAPve_g_L1_C0_1/1 -> SignalBusCreator/82(L1_C0)  "IMAPve_g_L1_C0"
  IMAPve_g_L1_C0/1 -> IMAPve_g_L1_C0_1/1
  IMAPve_g_R0_W_1/1 -> SignalBusCreator/81(R0_W)  "IMAPve_g_R0_W"
  IMAPve_g_R0_W/1 -> IMAPve_g_R0_W_1/1
  IMAPve_d_R0_Type_1/1 -> SignalBusCreator/80(R0_Type)  "IMAPve_d_R0_Type"
  IMAPve_d_R0_Type/1 -> IMAPve_d_R0_Type_1/1
  IMAPve_d_R0_Q_1/1 -> SignalBusCreator/79(R0_Q)  "IMAPve_d_R0_Q"
  IMAPve_d_R0_Q/1 -> IMAPve_d_R0_Q_1/1
  IMAPve_g_R0_VR_1/1 -> SignalBusCreator/78(R0_VR)  "IMAPve_g_R0_VR"
  IMAPve_g_R0_VR/1 -> IMAPve_g_R0_VR_1/1
  IMAPve_g_R0_C3_1/1 -> SignalBusCreator/77(R0_C3)  "IMAPve_g_R0_C3"
  IMAPve_g_R0_C3/1 -> IMAPve_g_R0_C3_1/1
  IMAPve_g_R0_C2_1/1 -> SignalBusCreator/76(R0_C2)  "IMAPve_g_R0_C2"
  IMAPve_g_R0_C2/1 -> IMAPve_g_R0_C2_1/1
  IMAPve_g_R0_C1_1/1 -> SignalBusCreator/75(R0_C1)  "IMAPve_g_R0_C1"
  IMAPve_g_R0_C1/1 -> IMAPve_g_R0_C1_1/1
  IMAPve_g_R0_C0_1/1 -> SignalBusCreator/74(R0_C0)  "IMAPve_g_R0_C0"
  IMAPve_g_R0_C0/1 -> IMAPve_g_R0_C0_1/1
  IMAPve_g_L0_W_1/1 -> SignalBusCreator/73(L0_W)  "IMAPve_g_L0_W"
  IMAPve_g_L0_W/1 -> IMAPve_g_L0_W_1/1
  IMAPve_d_L0_Type_1/1 -> SignalBusCreator/72(L0_Type)  "IMAPve_d_L0_Type"
  IMAPve_d_L0_Type/1 -> IMAPve_d_L0_Type_1/1
  IMAPve_d_L0_Q_1/1 -> SignalBusCreator/71(L0_Q)  "IMAPve_d_L0_Q"
  IMAPve_d_L0_Q/1 -> IMAPve_d_L0_Q_1/1
  IMAPve_g_L0_VR_1/1 -> SignalBusCreator/70(L0_VR)  "IMAPve_g_L0_VR"
  IMAPve_g_L0_VR/1 -> IMAPve_g_L0_VR_1/1
  IMAPve_g_L0_C3_1/1 -> SignalBusCreator/69(L0_C3)  "IMAPve_g_L0_C3"
  IMAPve_g_L0_C3/1 -> IMAPve_g_L0_C3_1/1
  IMAPve_g_L0_C2_1/1 -> SignalBusCreator/68(L0_C2)  "IMAPve_g_L0_C2"
  IMAPve_g_L0_C2/1 -> IMAPve_g_L0_C2_1/1
  IMAPve_g_L0_C1_1/1 -> SignalBusCreator/67(L0_C1)  "IMAPve_g_L0_C1"
  IMAPve_g_L0_C1/1 -> IMAPve_g_L0_C1_1/1
  IMAPve_g_L0_C0_1/1 -> SignalBusCreator/66(L0_C0)  "IMAPve_g_L0_C0"
  IMAPve_g_L0_C0/1 -> IMAPve_g_L0_C0_1/1
  IMAPva_d_obj_MotionStatus_1/1 -> SignalBusCreator/65(obj_MotionStatus)  "IMAPva_d_obj_MotionStatus"
  IMAPva_d_obj_MotionStatus/1 -> IMAPva_d_obj_MotionStatus_1/1
  IMAPva_d_obj_status_1/1 -> SignalBusCreator/64(obj_status)  "IMAPva_d_obj_status"
  IMAPva_d_obj_status/1 -> IMAPva_d_obj_status_1/1
  IMAPva_d_obj_lane_1/1 -> SignalBusCreator/63(obj_lane)  "IMAPva_d_obj_lane"
  IMAPva_d_obj_lane/1 -> IMAPva_d_obj_lane_1/1
  IMAPva_d_obj_class_1/1 -> SignalBusCreator/62(obj_class)  "IMAPva_d_obj_class"
  IMAPva_d_obj_class/1 -> IMAPva_d_obj_class_1/1
  IMAPva_g_obj_length_1/1 -> SignalBusCreator/61(obj_length)  "IMAPva_g_obj_length"
  IMAPva_g_obj_length/1 -> IMAPva_g_obj_length_1/1
  IMAPva_g_obj_width_1/1 -> SignalBusCreator/60(obj_width)  "IMAPva_g_obj_width"
  IMAPva_g_obj_width/1 -> IMAPva_g_obj_width_1/1
  IMAPva_g_obj_pos_var_xy_1/1 -> SignalBusCreator/59(obj_pos_var_xy)  "IMAPva_g_obj_pos_var_xy"
  IMAPva_g_obj_pos_var_xy/1 -> IMAPva_g_obj_pos_var_xy_1/1
  IMAPva_g_obj_pos_var_y_1/1 -> SignalBusCreator/58(obj_pos_var_y)  "IMAPva_g_obj_pos_var_y"
  IMAPva_g_obj_pos_var_y/1 -> IMAPva_g_obj_pos_var_y_1/1
  IMAPva_g_obj_pos_var_x_1/1 -> SignalBusCreator/57(obj_pos_var_x)  "IMAPva_g_obj_pos_var_x"
  IMAPva_g_obj_pos_var_x/1 -> IMAPva_g_obj_pos_var_x_1/1
  IMAPva_g_obj_acc_y_1/1 -> SignalBusCreator/56(obj_acc_y)  "IMAPva_g_obj_acc_y"
  IMAPva_g_obj_acc_y/1 -> IMAPva_g_obj_acc_y_1/1
  IMAPva_g_obj_acc_x_1/1 -> SignalBusCreator/55(obj_acc_x)  "IMAPva_g_obj_acc_x"
  IMAPva_g_obj_acc_x/1 -> IMAPva_g_obj_acc_x_1/1
  IMAPva_g_obj_vel_y_1/1 -> SignalBusCreator/54(obj_vel_y)  "IMAPva_g_obj_vel_y"
  IMAPva_g_obj_vel_y/1 -> IMAPva_g_obj_vel_y_1/1
  IMAPva_g_obj_vel_x_1/1 -> SignalBusCreator/53(obj_vel_x)  "IMAPva_g_obj_vel_x"
  IMAPva_g_obj_vel_x/1 -> IMAPva_g_obj_vel_x_1/1
  IMAPva_g_obj_pos_y_1/1 -> SignalBusCreator/52(obj_pos_y)  "IMAPva_g_obj_pos_y"
  IMAPva_g_obj_pos_y/1 -> IMAPva_g_obj_pos_y_1/1
  IMAPva_g_obj_pos_x_1/1 -> SignalBusCreator/51(obj_pos_x)  "IMAPva_g_obj_pos_x"
  IMAPva_g_obj_pos_x/1 -> IMAPva_g_obj_pos_x_1/1
  IMAPva_d_obj_id_1/1 -> SignalBusCreator/50(obj_id)  "IMAPva_d_obj_id"
  IMAPva_d_obj_id/1 -> IMAPva_d_obj_id_1/1
  IMAPve_d_obj_Num_1/1 -> SignalBusCreator/49(obj_Num)  "IMAPve_d_obj_Num"
  IMAPve_d_obj_Num/1 -> IMAPve_d_obj_Num_1/1
  IMAPve_d_Fusion_Status_1/1 -> SignalBusCreator/48(Fusion_Status)  "IMAPve_d_Fusion_Status"
  IMAPve_d_Fusion_Status/1 -> IMAPve_d_Fusion_Status_1/1
  IMAPve_d_Sensor_Status_1/1 -> SignalBusCreator/47(Sensor_Status)  "IMAPve_d_Sensor_Status"
  IMAPve_d_Sensor_Status/1 -> IMAPve_d_Sensor_Status_1/1
  IMAPve_d_Camera_Status_1/1 -> SignalBusCreator/46(Camera_Status)  "IMAPve_d_Camera_Status"
  IMAPve_d_Camera_Status/1 -> IMAPve_d_Camera_Status_1/1
  ADIAve_d_FuncFaultStatus_1/1 -> SignalBusCreator/45(ADIAve_d_FuncFaultStatus)  "ADIAve_d_FuncFaultStatus"
  ADIAve_d_FuncFaultStatus/1 -> ADIAve_d_FuncFaultStatus_1/1
  ADIAve_g_BSWFaultStatus_1/1 -> SignalBusCreator/44(ADIAve_g_BSWFaultStatus)  "ADIAve_g_BSWFaultStatus"
  ADIAve_g_BSWFaultStatus/1 -> ADIAve_g_BSWFaultStatus_1/1
  ADIAve_g_ASWFaultStatus_1/1 -> SignalBusCreator/43(ADIAve_g_ASWFaultStatus)  "ADIAve_g_ASWFaultStatus"
  ADIAve_g_ASWFaultStatus/1 -> ADIAve_g_ASWFaultStatus_1/1
  IMAPve_d_TCU_TCU_Available_1/1 -> SignalBusCreator/42(TCU_Available)  "IMAPve_d_TCU_TCU_Available"
  IMAPve_d_TCU_TCU_Available/1 -> IMAPve_d_TCU_TCU_Available_1/1
  IMAPve_d_TCU_Actual_Gear_1/1 -> SignalBusCreator/41(TCU_ActualGear)  "IMAPve_d_TCU_Actual_Gear"
  IMAPve_d_TCU_Actual_Gear/1 -> IMAPve_d_TCU_Actual_Gear_1/1
  IMAPve_g_EMS_RealPedal_1/1 -> SignalBusCreator/40(AccPedal_Pos)  "IMAPve_g_EMS_RealPedal"
  IMAPve_g_EMS_RealPedal/1 -> IMAPve_g_EMS_RealPedal_1/1
  IMAPve_d_BCM_HazardLamp_Switch_1/1 -> SignalBusCreator/39(BCM_Double_Light_Switch)  "IMAPve_d_BCM_HazardLamp_Switch"
  IMAPve_d_BCM_HazardLamp_Switch/1 -> IMAPve_d_BCM_HazardLamp_Switch_1/1
  IMAPve_d_BCM_RightTurn_Switch_1/1 -> SignalBusCreator/38(BCM_RightTurn_Switch)  "IMAPve_d_BCM_RightTurn_Switch"
  IMAPve_d_BCM_RightTurn_Switch/1 -> IMAPve_d_BCM_RightTurn_Switch_1/1
  IMAPve_d_BCM_LeftTurn_Switch_1/1 -> SignalBusCreator/37(BCM_LeftTurn_Switch)  "IMAPve_d_BCM_LeftTurn_Switch"
  IMAPve_d_BCM_LeftTurn_Switch/1 -> IMAPve_d_BCM_LeftTurn_Switch_1/1
  IMAPve_d_BCM_Right_Light_1/1 -> SignalBusCreator/36(BCM_Right_Light)  "IMAPve_d_BCM_Right_Light"
  IMAPve_d_BCM_Right_Light/1 -> IMAPve_d_BCM_Right_Light_1/1
  IMAPve_d_BCM_Left_Light_1/1 -> SignalBusCreator/35(BCM_Left_Light)  "IMAPve_d_BCM_Left_Light"
  IMAPve_d_BCM_Left_Light/1 -> IMAPve_d_BCM_Left_Light_1/1
  IMAPve_d_BCM_HazardLamp_1/1 -> SignalBusCreator/34(BCM_Double_Light)  "IMAPve_d_BCM_HazardLamp"
  IMAPve_d_BCM_HazardLamp/1 -> IMAPve_d_BCM_HazardLamp_1/1
  IMAPve_d_ESC_VehSpd_Valid_1/1 -> SignalBusCreator/33(ESC_VehSpd_Valid)  "IMAPve_d_ESC_VehSpd_Valid"
  IMAPve_d_ESC_VehSpd_Valid/1 -> IMAPve_d_ESC_VehSpd_Valid_1/1
  IMAPve_g_ESC_Brake_Press_1/1 -> SignalBusCreator/32(ESC_Brake_Press)  "IMAPve_g_ESC_Brake_Press"
  IMAPve_g_ESC_Brake_Press/1 -> IMAPve_g_ESC_Brake_Press_1/1
  IMAPve_d_ESC_LonAcc_Valid_1/1 -> SignalBusCreator/31(ESC_LonAcc_Valid)  "IMAPve_d_ESC_LonAcc_Valid"
  IMAPve_d_ESC_LonAcc_Valid/1 -> IMAPve_d_ESC_LonAcc_Valid_1/1
  IMAPve_g_ESC_LonAcc_1/1 -> SignalBusCreator/30(ESC_LonAcc)  "IMAPve_g_ESC_LonAcc"
  IMAPve_g_ESC_LonAcc/1 -> IMAPve_g_ESC_LonAcc_1/1
  IMAPve_g_ESC_VehSpd_1/1 -> SignalBusCreator/29(ESC_VehSpd)  "IMAPve_g_ESC_VehSpd"
  IMAPve_g_ESC_VehSpd/1 -> IMAPve_g_ESC_VehSpd_1/1
  IMAPve_g_ESC_UnYawRate_1/1 -> SignalBusCreator/28(ESC_UnYawRate)  "IMAPve_g_ESC_UnYawRate"
  IMAPve_g_ESC_UnYawRate/1 -> IMAPve_g_ESC_UnYawRate_1/1
  IMAPve_d_ESC_YawRate_Valid_1/1 -> SignalBusCreator/27(ESC_YawRate_Valid)  "IMAPve_d_ESC_YawRate_Valid"
  IMAPve_d_ESC_YawRate_Valid/1 -> IMAPve_d_ESC_YawRate_Valid_1/1
  IMAPve_g_ESC_YawRate_1/1 -> SignalBusCreator/26(ESC_YawRate)  "IMAPve_g_ESC_YawRate"
  IMAPve_g_ESC_YawRate/1 -> IMAPve_g_ESC_YawRate_1/1
  IMAPve_d_ESC_LatAcc_Valid_1/1 -> SignalBusCreator/25(ESC_LatAcc_Valid)  "IMAPve_d_ESC_LatAcc_Valid"
  IMAPve_d_ESC_LatAcc_Valid/1 -> IMAPve_d_ESC_LatAcc_Valid_1/1
  IMAPve_g_ESC_LatAcc_1/1 -> SignalBusCreator/24(ESC_LatAcc)  "IMAPve_g_ESC_LatAcc"
  IMAPve_g_ESC_LatAcc/1 -> IMAPve_g_ESC_LatAcc_1/1
  IMAPve_g_SW_Angle_Speed_1/1 -> SignalBusCreator/23(SW_Angle_Speed)  "IMAPve_g_SW_Angle_Speed"
  IMAPve_g_SW_Angle_Speed/1 -> IMAPve_g_SW_Angle_Speed_1/1
  IMAPve_g_SW_Angle_1/1 -> SignalBusCreator/22(SW_Angle)  "IMAPve_g_SW_Angle"
  IMAPve_g_SW_Angle/1 -> IMAPve_g_SW_Angle_1/1
  IMAPve_g_EPS_SteeringAngle_1/1 -> SignalBusCreator/21(EPS_SteeringAngle)  "IMAPve_g_EPS_SteeringAngle"
  IMAPve_g_EPS_SteeringAngle/1 -> IMAPve_g_EPS_SteeringAngle_1/1
  IMAPve_d_EPS_SteeringAngle_Flag_1/1 -> SignalBusCreator/20(EPS_SteeringAngle_Flag)  "IMAPve_d_EPS_SteeringAngle_Flag"
  IMAPve_d_EPS_SteeringAngle_Flag/1 -> IMAPve_d_EPS_SteeringAngle_Flag_1/1
  IMAPve_d_EPS_ESA_State_1/1 -> SignalBusCreator/19(EPS_ESA_State)  "IMAPve_d_EPS_ESA_State"
  IMAPve_d_EPS_ESA_State/1 -> IMAPve_d_EPS_ESA_State_1/1
  IMAPve_d_EPS_Driver_Override_1/1 -> SignalBusCreator/18(EPS_Driver_Override)  "IMAPve_d_EPS_Driver_Override"
  IMAPve_d_EPS_Driver_Override/1 -> IMAPve_d_EPS_Driver_Override_1/1
  IMAPve_d_EPS_Steer_Hold_State_1/1 -> SignalBusCreator/17(EPS_SWHold_State)  "IMAPve_d_EPS_Steer_Hold_State"
  IMAPve_d_EPS_Steer_Hold_State/1 -> IMAPve_d_EPS_Steer_Hold_State_1/1
  IMAPve_g_EPS_LKA_Current_1/1 -> SignalBusCreator/16(EPS_LKA_Current)  "IMAPve_g_EPS_LKA_Current"
  IMAPve_g_EPS_LKA_Current/1 -> IMAPve_g_EPS_LKA_Current_1/1
  IMAPve_d_EPS_TrqLim_State_1/1 -> SignalBusCreator/15(EPS_TrqLim_State)  "IMAPve_d_EPS_TrqLim_State"
  IMAPve_d_EPS_TrqLim_State/1 -> IMAPve_d_EPS_TrqLim_State_1/1
  IMAPve_d_SWS_Failure_Status_1/1 -> SignalBusCreator/14(SWS_Failure_Status)  "IMAPve_d_SWS_Failure_Status"
  IMAPve_d_SWS_Failure_Status/1 -> IMAPve_d_SWS_Failure_Status_1/1
  IMAPve_d_SAS_Trim_State_1/1 -> SignalBusCreator/13(SAS_Trim_State)  "IMAPve_d_SAS_Trim_State"
  IMAPve_d_SAS_Trim_State/1 -> IMAPve_d_SAS_Trim_State_1/1
  IMAPve_d_SAS_Clb_State_1/1 -> SignalBusCreator/12(SAS_Clb_State)  "IMAPve_d_SAS_Clb_State"
  IMAPve_d_SAS_Clb_State/1 -> IMAPve_d_SAS_Clb_State_1/1
  IMAPve_d_EPS_Trq_State_1/1 -> SignalBusCreator/11(EPS_Trq_State)  "IMAPve_d_EPS_Trq_State"
  IMAPve_d_EPS_Trq_State/1 -> IMAPve_d_EPS_Trq_State_1/1
  IMAPve_g_EPS_SW_Trq_1/1 -> SignalBusCreator/10(EPS_SW_Trq)  "IMAPve_g_EPS_SW_Trq"
  IMAPve_g_EPS_SW_Trq/1 -> IMAPve_g_EPS_SW_Trq_1/1
  IMAPve_d_EPS_LKA_State_1/1 -> SignalBusCreator/9(EPS_LKA_State)  "IMAPve_d_EPS_LKA_State"
  IMAPve_d_EPS_LKA_State/1 -> IMAPve_d_EPS_LKA_State_1/1
  IMAPve_d_MP5_Work_State_1/1 -> SignalBusCreator/8(MP5_Work_State)  "IMAPve_d_MP5_Work_State"
  IMAPve_d_MP5_Work_State/1 -> IMAPve_d_MP5_Work_State_1/1
  IMAPve_d_APA_AutoPark_WorkSt_1/1 -> SignalBusCreator/7(APA_AutoPark_WorkSt)  "IMAPve_d_APA_AutoPark_WorkSt"
  IMAPve_d_APA_AutoPark_WorkSt/1 -> IMAPve_d_APA_AutoPark_WorkSt_1/1
  IMAPve_d_ELK_Switch_1/1 -> SignalBusCreator/6(ELK_Switch)  "IMAPve_d_ELK_Switch"
  IMAPve_d_ELK_Switch/1 -> IMAPve_d_ELK_Switch_1/1
  IMAPve_d_LDW_Warn_Mode_1/1 -> SignalBusCreator/5(LDW_Warn_Mode)  "IMAPve_d_LDW_Warn_Mode"
  IMAPve_d_LDW_Warn_Mode/1 -> IMAPve_d_LDW_Warn_Mode_1/1
  IMAPve_d_LKA_Mode_1/1 -> SignalBusCreator/4(LKA_Mode)  "IMAPve_d_LKA_Mode"
  IMAPve_d_LKA_Mode/1 -> IMAPve_d_LKA_Mode_1/1
  IMAPve_d_LKA_Main_Switch_1/1 -> SignalBusCreator/3(LKA_Main_Switch)  "IMAPve_d_LKA_Main_Switch"
  IMAPve_d_LKA_Main_Switch/1 -> IMAPve_d_LKA_Main_Switch_1/1
  FDMMve_d_ElkFcnConf_1/1 -> SignalBusCreator/2(ElkFcnConf)  "FDMMve_d_ElkFcnConf"
  FDMMve_d_ElkFcnConf/1 -> FDMMve_d_ElkFcnConf_1/1
  FDMMve_d_LkaFcnConf_1/1 -> SignalBusCreator/1(LkaFcnConf)  "FDMMve_d_LkaFcnConf"
  FDMMve_d_LkaFcnConf/1 -> FDMMve_d_LkaFcnConf_1/1

== system LKAS_AutoSave_DF_20220421_1805_SW62/LKAS/LL ==
  bsInInfo : Inport
  bsLLClb : Inport  Port=2
  Bus Selector : BusSelector  OutputSignals=bsMP5Info.LKA_Main_Switch
  Fault_Diagnostic : Subsystem
  Human Machine Interface (HMI) : Subsystem
  LL Inputs Mapping : Subsystem
  LLOn : Subsystem
  LLOut : Subsystem
  Terminator : Terminator
  Version : Constant  Value=220421  OutMin=20410  OutMax=220630  OutDataTypeStr=single
  LL_bsLLOut : Outport
      settings: AttributesFormatString=Disable Action: %<OutputWhenDisabled>
  tag scope: LLMon=global
  wires:
  [bsLLClb] -> Human Machine Interface (HMI)/4(HMI_bsLLClb)
  [LLOn_bsLDWWarnInfo] -> Human Machine Interface (HMI)/3(HMI_bsLDWWarnInfo)
  [LLOn_bsLLState] -> Human Machine Interface (HMI)/2(HMI_bsLLState)
  [bsInfo] -> Human Machine Interface (HMI)/1(HMI_bsInfo)
  Human Machine Interface (HMI)/1(HMI_LDWLKA) -> [HMI_bsLLHMI]  "bsLLHMI"
  [bsLLClb] -> LL Inputs Mapping/2(bsLLClb)
  [bsFaultStatus] -> LLOn/3(bsSignalFault)
  [bsLLClb] -> LLOn/2(bsLLClb)
  [bsInfo] -> LLOn/1(bsInInfo), Bus Selector/1
  [bsInInfo] -> LL Inputs Mapping/1(bsInInfo)
  LL Inputs Mapping/1(bsInfo) -> [bsInfo]
  [bsInInfo] -> Fault_Diagnostic/1(bsInInfo)
  Fault_Diagnostic/1(bsFaultStatus) -> [bsFaultStatus]
  LLOn/5(LLMon) -> [LLMon]
  LLOn/4(M) -> [LLOn_M]
  LLOn/3(phiSWACmd) -> [LLOn_phiSWACmd]
  LLOn/1(bsLLState) -> [LLOn_bsLLState]
  bsLLClb/1 -> [bsLLClb]
  LLOn/2(LDW_Flag) -> [LLOn_bsLDWWarnInfo]
  Version/1 -> Terminator/1  "ob_LKA_Version"
  bsInInfo/1 -> [bsInInfo]
  Bus Selector/1 -> LLOn/Enable  "<LKA_Main_Switch>"
  [HMI_bsLLHMI] -> LLOut/3(LLOut_bsLLHMI)
  LLOut/1(LL_bsLLOut) -> LL_bsLLOut/1
  [LLOn_bsLLState] -> LLOut/1(LLOut_bsLLState)
  [LLOn_M] -> LLOut/4(LLOut_M)
  [bsInfo] -> LLOut/5(LLOut_bsInfo)
  [LLOn_phiSWACmd] -> LLOut/2(LLOut_phiSWACmd)

== system LKAS_AutoSave_DF_20220421_1805_SW62/LKAS/LLClb ==
  Bus Creator : BusCreator  Inputs=4
  ConstantClb : Subsystem
  LDWClb : Subsystem
  LKAClb : Subsystem
  LLSMConClb : Subsystem
  LLClb_bsLLClb : Outport
  wires:
  LKAClb/1(LKAClb) -> Bus Creator/3  "bsLKAClb"
  LDWClb/1(LDWClb) -> Bus Creator/2  "bsLDWClb"
  Bus Creator/1 -> LLClb_bsLLClb/1  "bsLLClb"
  LLSMConClb/1(LLSMConClb) -> Bus Creator/1  "bsLLSMConClb"
  ConstantClb/1(ConstantClb) -> Bus Creator/4  "bsConstantClb"
